simulink model "Simulation_Model_2"  (Simulink 10.1)
settings: Solver=VariableStepAuto  StartTime=0.0  StopTime=10.0  RelTol=1e-3
settings Model: Creator=Dravius  LastModifiedBy=Roma
settings DataIOCC: SaveFormat=Dataset
settings OptimizationCC: LifeSpan=auto
settings DebuggingCC: UnderspecifiedInitializationDetection=Simplified  MergeDetectMultiDrivingBlocksExec=error  SFUnexpectedBacktrackingDiag=error  SFNoUnconditionalDefaultTransitionDiag=error  SFExecutionAtInitializationDiag=warning
settings HardwareCC: ProdBitPerPointer=64  ProdBitPerSizeT=64  ProdBitPerPtrDiffT=64  ProdLargestAtomicFloat=Float  ProdIntDivRoundTo=Zero  ProdEndianess=LittleEndian  ProdWordSize=64  ProdHWDeviceType=Intel->x86-64 (Windows64)
settings ModelReferenceCC: PropagateSignalLabelsOutOfModel=on
settings SFSimCC: SimUseLocalCustomCode=on
settings RTWCC: RTWUseLocalCustomCode=on
settings CodeAppCC: StateflowObjectComments=off
settings GRTTargetCC: TargetLangStandard=C99 (ISO)  CombineOutputUpdateFcns=on  GRTInterface=off
settings ConfigComp: CovMetricSettings=dwe  CovHtmlReporting=off  CovSaveCumulativeToWorkspaceVar=off  CovSaveSingleToWorkspaceVar=off  CovExternalEMLEnable=on

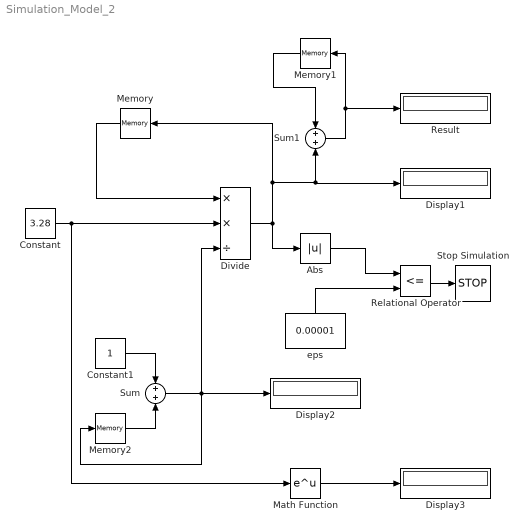
== system Simulation_Model_2 ==
  Abs : Abs
  Constant : Constant  Value=3.28
  Constant1 : Constant
  Display1 : Display
  Display2 : Display
  Display3 : Display
  Divide : Product  Inputs=**/
  Math Function : Math  SignedPower=on  SaturateOnIntegerOverflow=on
  Memory : Memory  InitialCondition=1
  Memory1 : Memory  InitialCondition=1
  Memory2 : Memory
  Relational Operator : RelationalOperator  Operator=<=  OutDataTypeStr=boolean  RndMeth=Simplest
  Result : Display
  Stop Simulation : Stop
  Sum : Sum
  Sum1 : Sum
  eps : Constant  Value=0.00001
  wires:
  Constant/1 -> Math Function/1, Divide/2
  Constant1/1 -> Sum/1
  Memory2/1 -> Sum/2
  Sum/1 -> Divide/3, Display2/1, Memory2/1
  Memory/1 -> Divide/1
  Divide/1 -> Memory/1, Display1/1, Sum1/2, Abs/1
  Sum1/1 -> Memory1/1, Result/1
  Memory1/1 -> Sum1/1
  Abs/1 -> Relational Operator/1
  Relational Operator/1 -> Stop Simulation/1
  eps/1 -> Relational Operator/2
  Math Function/1 -> Display3/1
